simulink model "lab5_host"  (R2021b)
settings: Solver=ode1  StartTime=0.0  StopTime=inf  FixedStep=1e-3  RelTol=1e-3
InitFcn:
  | X_to_L = 1/(20*2*pi);
libraries: slrealtimeutilitieslib x1, slrealtimeiplib x1
settings Model: Creator=tcraddoc  LastModifiedBy=wasynczu
settings SolverCC: AlgebraicLoopSolver=TrustRegion
settings DataIOCC: ReturnWorkspaceOutputs=off
settings DebuggingCC: SFMachineParentedDataDiag=warning  ArithmeticOperatorsInVariantConditions=warning
settings SFSimCC: SimUseLocalCustomCode=off  CustomCodeUndefinedFunction=UseInterfaceOnly
settings RTWCC: RTWUseLocalCustomCode=off
settings CodeAppCC: StateflowObjectComments=on

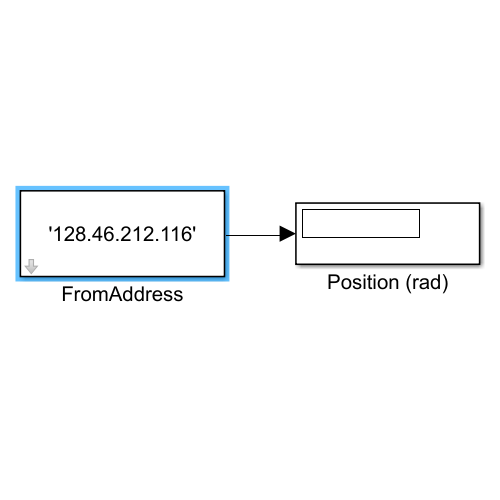
[thumbnail: Simulink's stored preview of the top-level diagram]
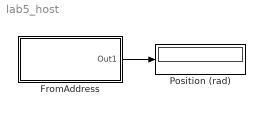
== system lab5_host ==
  FromAddress : Subsystem  mask{fromIPAddress='128.46.212.116'}
      mask prompts: fromIPAddress "From IP Address"
      mask Display: disp((get_param(gcb,'fromIPAddress')))
  Position (rad) : Display
  wires:
  FromAddress/1(Out1) -> Position (rad)/1

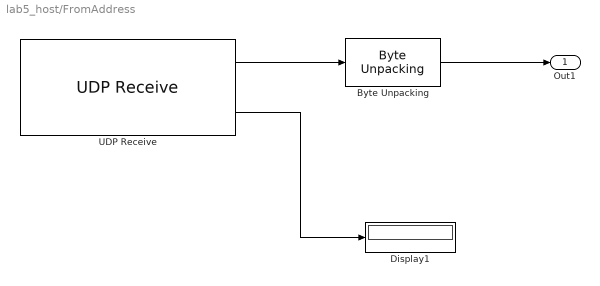
== system lab5_host/FromAddress ==
  Byte Unpacking : slrealtimeutilitieslib/Byte Unpacking  MaskUnpackedDataTypes={['double']}  MaskUnpackedDataSizes={[1]}  MaskAlignment=1
      settings: SourceProductBaseCode=XP
  Display1 : Display
  UDP Receive : slrealtimeiplib/UDP Receive  useHostTargetConn=on  ipAddress=128.46.212.188  localPort=34  rcvWidth=8  rcvFmAny=off  fmAddress=fromIPAddress  sampleTime=1e-3
      settings: SourceProductBaseCode=XP
  Out1 : Outport
  wires:
  Byte Unpacking/1 -> Out1/1
  UDP Receive/2 -> Display1/1
  UDP Receive/1 -> Byte Unpacking/1
